simulink model "gm_interlock_deadtime"  (R2020b)
settings: Solver=FixedStepDiscrete  StartTime=0.0  StopTime=0.01  RelTol=1e-3
libraries: hdlmdlgenlib x12, simulink x6, hdlsllib x6, eePwmGeneratorTwoLevel x1, powerlib_meascontrol x1
settings Model: Creator=ts  LastModifiedBy=ts
settings DataIOCC: LimitDataPoints=on  SaveOutput=off  SaveTime=off
settings OptimizationCC: BlockReduction=off  ConditionallyExecuteInputs=off  DefaultParameterBehavior=Inlined  LifeSpan=inf
settings DebuggingCC: AlgebraicLoopMsg=error  InheritedTsInSrcMsg=none  SingleTaskRateTransMsg=error  AllowSymbolicDim=off  StrictBusMsg=ErrorOnBusTreatedAsVector  SFUnexpectedBacktrackingDiag=warning  SFNoUnconditionalDefaultTransitionDiag=warning  SFExecutionAtInitializationDiag=none  ArithmeticOperatorsInVariantConditions=warning
settings HardwareCC: ProdBitPerPointer=32  ProdBitPerSizeT=32  ProdBitPerPtrDiffT=32  ProdLargestAtomicFloat=None  ProdIntDivRoundTo=Undefined  ProdEndianess=Unspecified  ProdWordSize=32  ProdHWDeviceType=ASIC/FPGA->ASIC/FPGA  ProdEqTarget=off
settings SFSimCC: SimUseLocalCustomCode=off  CustomCodeUndefinedFunction=UseInterfaceOnly
settings RTWCC: RTWUseLocalCustomCode=off
settings CodeAppCC: StateflowObjectComments=on
settings GRTTargetCC: TargetLangStandard=C89/C90 (ANSI)
settings ConfigComp: CovScope=ReferencedModels  CovMetricSettings=dw  CovSaveCumulativeToWorkspaceVar=on  CovSaveSingleToWorkspaceVar=on  CovExternalEMLEnable=off  CovSFcnEnable=off

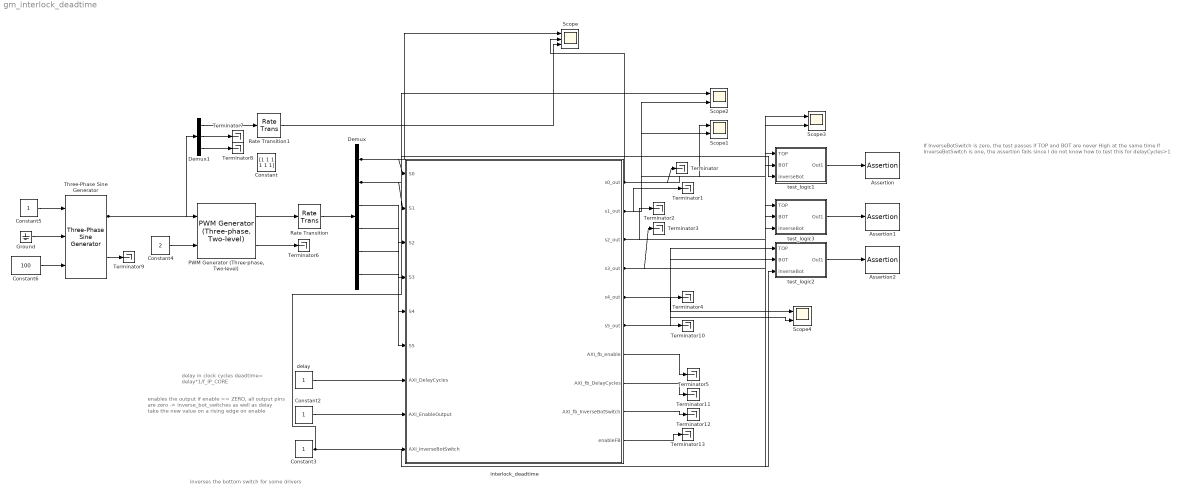
== system gm_interlock_deadtime ==
  note: delay in clock cycles
      | deadtime= delay*1/f_IP_CORE
  note: inverses the bottom switch for some drivers
  note: enables the output
      | if enable == ZERO, all output pins are zero
      |
      | -> inverse_bot_switches as well as delay take the
      | new value on a rising edge on enable
  note: If InverseBotSwitch is zero, the test passes if TOP and BOT are never High at the same time
      | If InverseBotSwitch is one, the assertion fails since I do not know how to test this for delayCycles>1
  Assertion : Assertion
  Assertion1 : Assertion
  Assertion2 : Assertion
  Constant : Constant  Value=[1 1 1 1 1 1]  OutDataTypeStr=boolean
  Constant2 : Constant  OutDataTypeStr=boolean  SampleTime=1/100e6
  Constant3 : Constant  OutDataTypeStr=boolean  SampleTime=1/100e6
  Constant4 : Constant  Value=2  SampleTime=-1
  Constant5 : Constant  SampleTime=-1
  Constant6 : Constant  Value=100  SampleTime=-1
  Demux : Demux  Outputs=6
  Demux1 : Demux  Outputs=3
  Ground : Ground
  "PWM Generator (Three-phase, Two-level)" : eePwmGeneratorTwoLevel/PWM Generator (Three-phase, Two-level)  PWMMode=Continuous PWM (CPWM)  CPWMMode=SPWM: sinusoidal PWM  DPWMMode=60 DPWM: 60 degree discontinuous PWM  fsw=10e3  Ts=1/(100*100e3)
      settings: SourceProductBaseCode=PS
  Rate Transition : RateTransition  OutPortSampleTime=1/100e6
  Rate Transition1 : RateTransition  OutPortSampleTime=1/100e6
  Scope : Scope  NumInputPorts=3
  Scope{1..4} (4 alike) : Scope  NumInputPorts=2
  Terminator{,1..13} (14 alike) : Terminator
  Three-Phase Sine Generator : powerlib_meascontrol/Pulse & Signal Generators/Three-Phase Sine Generator  Ts=1/100e3
      settings: SourceProductBaseCode=PS
  delay : Constant  OutDataTypeStr=fixdt(0,10,0)  SampleTime=1/100e6
  interlock_deadtime : Subsystem  TreatAsAtomicUnit=on
  test_logic1 : Subsystem
  test_logic2 : Subsystem
  test_logic3 : Subsystem
  wires:
  delay/1 -> interlock_deadtime/7(AXI_DelayCycles)
  "PWM Generator (Three-phase, Two-level)"/1 -> Rate Transition/1
  Rate Transition/1 -> Demux/1
  test_logic1/1(Out1) -> Assertion/1
  test_logic2/1(Out1) -> Assertion2/1
  test_logic3/1(Out1) -> Assertion1/1
  interlock_deadtime/10(enableFB) -> Terminator13/1
  interlock_deadtime/9(AXI_fb_InverseBotSwitch) -> Terminator12/1
  interlock_deadtime/8(AXI_fb_DelayCycles) -> Terminator11/1
  interlock_deadtime/7(AXI_fb_enable) -> Terminator5/1
  interlock_deadtime/6(s5_out) -> Terminator10/1, test_logic2/2(BOT), Scope4/2
  Ground/1 -> Three-Phase Sine Generator/2
  Three-Phase Sine Generator/2 -> Terminator9/1
  Demux1/3 -> Terminator8/1
  Demux1/2 -> Terminator7/1
  "PWM Generator (Three-phase, Two-level)"/2 -> Terminator6/1
  Constant3/1 -> test_logic1/3(inverseBot), test_logic3/3(inverseBot), test_logic2/3(inverseBot), interlock_deadtime/9(AXI_InverseBotSwitch)
  Rate Transition1/1 -> Scope/3
  Demux1/1 -> Rate Transition1/1
  Demux/6 -> interlock_deadtime/6(S5)
  Demux/5 -> interlock_deadtime/5(S4)
  Demux/4 -> interlock_deadtime/4(S3)
  Demux/3 -> interlock_deadtime/3(S2)
  Demux/2 -> interlock_deadtime/2(S1), Scope2/1
  Demux/1 -> interlock_deadtime/1(S0), Scope/1
  Constant6/1 -> Three-Phase Sine Generator/3
  Constant5/1 -> Three-Phase Sine Generator/1
  Three-Phase Sine Generator/1 -> "PWM Generator (Three-phase, Two-level)"/1, Demux1/1
  Constant4/1 -> "PWM Generator (Three-phase, Two-level)"/2
  interlock_deadtime/5(s4_out) -> Terminator4/1, test_logic2/1(TOP), Scope4/1
  interlock_deadtime/4(s3_out) -> Terminator3/1, test_logic3/2(BOT), Scope3/2
  interlock_deadtime/3(s2_out) -> Terminator2/1, test_logic3/1(TOP), Scope3/1
  interlock_deadtime/2(s1_out) -> Terminator1/1, test_logic1/2(BOT), Scope2/2, Scope1/2
  interlock_deadtime/1(s0_out) -> Scope1/1, Terminator/1, test_logic1/1(TOP), Scope/2
  Constant2/1 -> interlock_deadtime/8(AXI_EnableOutput)

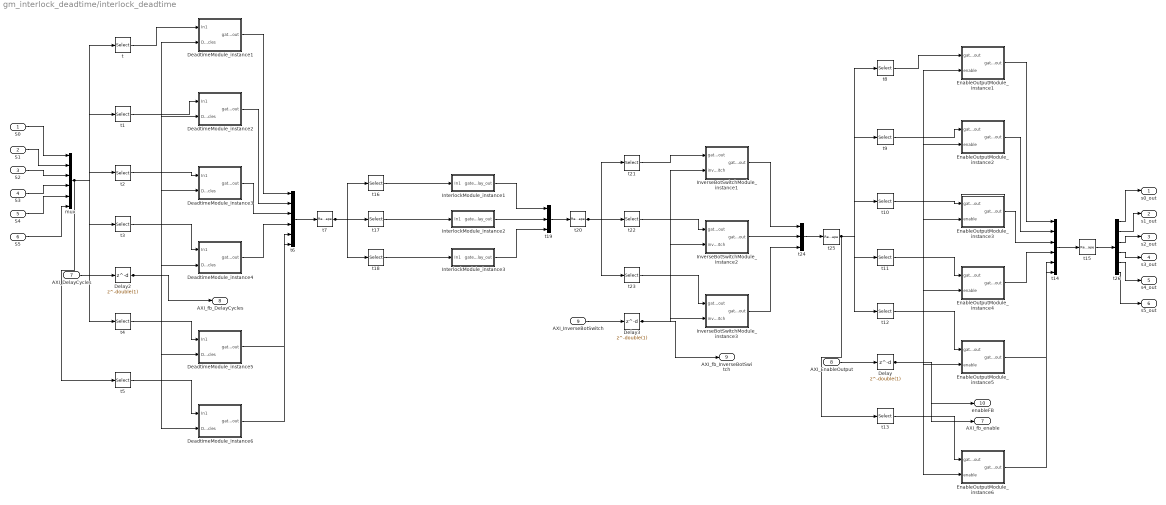
== system gm_interlock_deadtime/interlock_deadtime ==
  S0 : Inport  OutDataTypeStr=boolean  PortDimensions=1  SampleTime=1e-08
  S1 : Inport  Port=2  OutDataTypeStr=boolean  PortDimensions=1  SampleTime=1e-08
  S2 : Inport  Port=3  OutDataTypeStr=boolean  PortDimensions=1  SampleTime=1e-08
  S3 : Inport  Port=4  OutDataTypeStr=boolean  PortDimensions=1  SampleTime=1e-08
  S4 : Inport  Port=5  OutDataTypeStr=boolean  PortDimensions=1  SampleTime=1e-08
  S5 : Inport  Port=6  OutDataTypeStr=boolean  PortDimensions=1  SampleTime=1e-08
  AXI_DelayCycles : Inport  Port=7  OutDataTypeStr=fixdt(0, 10, 0)  PortDimensions=1  SampleTime=1e-08
  AXI_EnableOutput : Inport  Port=8  OutDataTypeStr=boolean  PortDimensions=1  SampleTime=1e-08
  AXI_InverseBotSwitch : Inport  Port=9  OutDataTypeStr=boolean  PortDimensions=1  SampleTime=1e-08
  DeadtimeModule_instance1 : Subsystem
  DeadtimeModule_instance2 : Subsystem
  DeadtimeModule_instance3 : Subsystem
  DeadtimeModule_instance4 : Subsystem
  DeadtimeModule_instance5 : Subsystem
  DeadtimeModule_instance6 : Subsystem
  Delay : Delay  DelayLength=double(1)  InitialCondition=0  SampleTime=1e-08
  Delay2 : Delay  DelayLength=double(1)  InitialCondition=0  SampleTime=1e-08
  Delay3 : Delay  DelayLength=double(1)  InitialCondition=0  SampleTime=1e-08
  EnableOutputModule_instance1 : Subsystem
  EnableOutputModule_instance2 : Subsystem
  EnableOutputModule_instance3 : Subsystem
  EnableOutputModule_instance4 : Subsystem
  EnableOutputModule_instance5 : Subsystem
  EnableOutputModule_instance6 : Subsystem
  InterlockModule_instance1 : Subsystem
  InterlockModule_instance2 : Subsystem
  InterlockModule_instance3 : Subsystem
  InverseBotSwitchModule_instance1 : Subsystem
  InverseBotSwitchModule_instance2 : Subsystem
  InverseBotSwitchModule_instance3 : Subsystem
  mux : Mux  Inputs=6
  t : Selector  SampleTime=1e-08  IndexOptions=Index vector (dialog)  Indices=double(1)  OutputSizes=1
  t1 : Selector  SampleTime=1e-08  IndexOptions=Index vector (dialog)  Indices=double(2)  OutputSizes=1
  t10 : Selector  SampleTime=1e-08  IndexOptions=Index vector (dialog)  Indices=double(3)  OutputSizes=1
  t11 : Selector  SampleTime=1e-08  IndexOptions=Index vector (dialog)  Indices=double(4)  OutputSizes=1
  t12 : Selector  SampleTime=1e-08  IndexOptions=Index vector (dialog)  Indices=double(5)  OutputSizes=1
  t13 : Selector  SampleTime=1e-08  IndexOptions=Index vector (dialog)  Indices=double(6)  OutputSizes=1
  t14 : Concatenate  NumInputs=6
  t{7,15,20,25} (4 alike) : Reshape
  t16 : Selector  SampleTime=1e-08  IndexOptions=Index vector (dialog)  Indices=double([1 2])  OutputSizes=1
  t17 : Selector  SampleTime=1e-08  IndexOptions=Index vector (dialog)  Indices=double([3 4])  OutputSizes=1
  t18 : Selector  SampleTime=1e-08  IndexOptions=Index vector (dialog)  Indices=double([5 6])  OutputSizes=1
  t19 : Concatenate  NumInputs=3
  t2 : Selector  SampleTime=1e-08  IndexOptions=Index vector (dialog)  Indices=double(3)  OutputSizes=1
  t21 : Selector  SampleTime=1e-08  IndexOptions=Index vector (dialog)  Indices=double([1 2])  OutputSizes=1
  t22 : Selector  SampleTime=1e-08  IndexOptions=Index vector (dialog)  Indices=double([3 4])  OutputSizes=1
  t23 : Selector  SampleTime=1e-08  IndexOptions=Index vector (dialog)  Indices=double([5 6])  OutputSizes=1
  t24 : Concatenate  NumInputs=3
  t26 : Demux  Outputs=6
  t3 : Selector  SampleTime=1e-08  IndexOptions=Index vector (dialog)  Indices=double(4)  OutputSizes=1
  t4 : Selector  SampleTime=1e-08  IndexOptions=Index vector (dialog)  Indices=double(5)  OutputSizes=1
  t5 : Selector  SampleTime=1e-08  IndexOptions=Index vector (dialog)  Indices=double(6)  OutputSizes=1
  t6 : Concatenate  NumInputs=6
  t8 : Selector  SampleTime=1e-08  IndexOptions=Index vector (dialog)  Indices=double(1)  OutputSizes=1
  t9 : Selector  SampleTime=1e-08  IndexOptions=Index vector (dialog)  Indices=double(2)  OutputSizes=1
  s0_out : Outport  VectorParamsAs1DForOutWhenUnconnected=off
  s1_out : Outport  Port=2  VectorParamsAs1DForOutWhenUnconnected=off
  s2_out : Outport  Port=3  VectorParamsAs1DForOutWhenUnconnected=off
  s3_out : Outport  Port=4  VectorParamsAs1DForOutWhenUnconnected=off
  s4_out : Outport  Port=5  VectorParamsAs1DForOutWhenUnconnected=off
  s5_out : Outport  Port=6  VectorParamsAs1DForOutWhenUnconnected=off
  AXI_fb_enable : Outport  Port=7  VectorParamsAs1DForOutWhenUnconnected=off
  AXI_fb_DelayCycles : Outport  Port=8  VectorParamsAs1DForOutWhenUnconnected=off
  AXI_fb_InverseBotSwitch : Outport  Port=9  VectorParamsAs1DForOutWhenUnconnected=off
  enableFB : Outport  Port=10  VectorParamsAs1DForOutWhenUnconnected=off
  wires:
  S0/1 -> mux/1
  S1/1 -> mux/2
  S2/1 -> mux/3
  S3/1 -> mux/4
  S4/1 -> mux/5
  S5/1 -> mux/6
  AXI_DelayCycles/1 -> Delay2/1
  AXI_EnableOutput/1 -> Delay/1
  AXI_InverseBotSwitch/1 -> Delay3/1
  t7/1 -> t18/1, t17/1, t16/1
  Delay/1 -> EnableOutputModule_instance6/2(enable), EnableOutputModule_instance5/2(enable), EnableOutputModule_instance4/2(enable), EnableOutputModule_instance3/2(enable), EnableOutputModule_instance2/2(enable), EnableOutputModule_instance1/2(enable), AXI_fb_enable/1, enableFB/1
  Delay2/1 -> DeadtimeModule_instance6/2(DelayCycles), DeadtimeModule_instance5/2(DelayCycles), DeadtimeModule_instance4/2(DelayCycles), DeadtimeModule_instance3/2(DelayCycles), DeadtimeModule_instance2/2(DelayCycles), DeadtimeModule_instance1/2(DelayCycles), AXI_fb_DelayCycles/1
  Delay3/1 -> InverseBotSwitchModule_instance3/2(inverse_bottom_switch), InverseBotSwitchModule_instance2/2(inverse_bottom_switch), InverseBotSwitchModule_instance1/2(inverse_bottom_switch), AXI_fb_InverseBotSwitch/1
  t15/1 -> t26/1
  t20/1 -> t23/1, t22/1, t21/1
  t25/1 -> t13/1, t12/1, t11/1, t10/1, t9/1, t8/1
  mux/1 -> t5/1, t4/1, t3/1, t2/1, t1/1, t/1
  t/1 -> DeadtimeModule_instance1/1(In1)
  t1/1 -> DeadtimeModule_instance2/1(In1)
  t2/1 -> DeadtimeModule_instance3/1(In1)
  t3/1 -> DeadtimeModule_instance4/1(In1)
  t4/1 -> DeadtimeModule_instance5/1(In1)
  t5/1 -> DeadtimeModule_instance6/1(In1)
  t6/1 -> t7/1
  DeadtimeModule_instance1/1(gate_delay_out) -> t6/1
  DeadtimeModule_instance2/1(gate_delay_out) -> t6/2
  DeadtimeModule_instance3/1(gate_delay_out) -> t6/3
  DeadtimeModule_instance4/1(gate_delay_out) -> t6/4
  DeadtimeModule_instance5/1(gate_delay_out) -> t6/5
  DeadtimeModule_instance6/1(gate_delay_out) -> t6/6
  t8/1 -> EnableOutputModule_instance1/1(gate_delay_out)
  t9/1 -> EnableOutputModule_instance2/1(gate_delay_out)
  t10/1 -> EnableOutputModule_instance3/1(gate_delay_out)
  t11/1 -> EnableOutputModule_instance4/1(gate_delay_out)
  t12/1 -> EnableOutputModule_instance5/1(gate_delay_out)
  t13/1 -> EnableOutputModule_instance6/1(gate_delay_out)
  t14/1 -> t15/1
  EnableOutputModule_instance1/1(gate_enable_out) -> t14/1
  EnableOutputModule_instance2/1(gate_enable_out) -> t14/2
  EnableOutputModule_instance3/1(gate_enable_out) -> t14/3
  EnableOutputModule_instance4/1(gate_enable_out) -> t14/4
  EnableOutputModule_instance5/1(gate_enable_out) -> t14/5
  EnableOutputModule_instance6/1(gate_enable_out) -> t14/6
  t16/1 -> InterlockModule_instance1/1(In1)
  t17/1 -> InterlockModule_instance2/1(In1)
  t18/1 -> InterlockModule_instance3/1(In1)
  t19/1 -> t20/1
  InterlockModule_instance1/1(gate_delay_out) -> t19/1
  InterlockModule_instance2/1(gate_delay_out) -> t19/2
  InterlockModule_instance3/1(gate_delay_out) -> t19/3
  t21/1 -> InverseBotSwitchModule_instance1/1(gate_delay_out)
  t22/1 -> InverseBotSwitchModule_instance2/1(gate_delay_out)
  t23/1 -> InverseBotSwitchModule_instance3/1(gate_delay_out)
  t24/1 -> t25/1
  InverseBotSwitchModule_instance1/1(gate_enable_out) -> t24/1
  InverseBotSwitchModule_instance2/1(gate_enable_out) -> t24/2
  InverseBotSwitchModule_instance3/1(gate_enable_out) -> t24/3
  t26/1 -> s0_out/1
  t26/2 -> s1_out/1
  t26/3 -> s2_out/1
  t26/4 -> s3_out/1
  t26/5 -> s4_out/1
  t26/6 -> s5_out/1

== system gm_interlock_deadtime/test_logic1 ==
  TOP : Inport
  BOT : Inport  Port=2
  inverseBot : Inport  Port=3
  AND : Logic  IconShape=distinctive  AllPortsSameDT=off  OutDataTypeStr=boolean
  Constant : Constant
  NOT : Logic  Operator=NOT  IconShape=distinctive  AllPortsSameDT=off  OutDataTypeStr=boolean
  Switch : Switch  Criteria=u2 ~= 0
  Out1 : Outport
  wires:
  BOT/1 -> AND/2
  TOP/1 -> AND/1
  NOT/1 -> Switch/3
  inverseBot/1 -> Switch/2
  AND/1 -> NOT/1
  Switch/1 -> Out1/1
  Constant/1 -> Switch/1

== system gm_interlock_deadtime/test_logic2 ==
  TOP : Inport
  BOT : Inport  Port=2
  inverseBot : Inport  Port=3
  AND : Logic  IconShape=distinctive  AllPortsSameDT=off  OutDataTypeStr=boolean
  Constant : Constant
  NOT : Logic  Operator=NOT  IconShape=distinctive  AllPortsSameDT=off  OutDataTypeStr=boolean
  Switch : Switch  Criteria=u2 ~= 0
  Out1 : Outport
  wires:
  Constant/1 -> Switch/1
  Switch/1 -> Out1/1
  AND/1 -> NOT/1
  inverseBot/1 -> Switch/2
  NOT/1 -> Switch/3
  TOP/1 -> AND/1
  BOT/1 -> AND/2

== system gm_interlock_deadtime/test_logic3 ==
  TOP : Inport
  BOT : Inport  Port=2
  inverseBot : Inport  Port=3
  AND : Logic  IconShape=distinctive  AllPortsSameDT=off  OutDataTypeStr=boolean
  Constant : Constant
  NOT : Logic  Operator=NOT  IconShape=distinctive  AllPortsSameDT=off  OutDataTypeStr=boolean
  Switch : Switch  Criteria=u2 ~= 0
  Out1 : Outport
  wires:
  BOT/1 -> AND/2
  TOP/1 -> AND/1
  NOT/1 -> Switch/3
  inverseBot/1 -> Switch/2
  AND/1 -> NOT/1
  Switch/1 -> Out1/1
  Constant/1 -> Switch/1

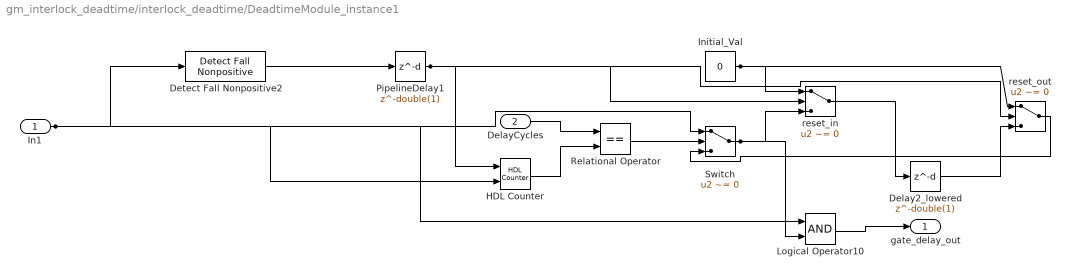
== system gm_interlock_deadtime/interlock_deadtime/DeadtimeModule_instance1 ==
  In1 : Inport  OutDataTypeStr=boolean  PortDimensions=1  SampleTime=1e-08
  DelayCycles : Inport  Port=2  OutDataTypeStr=fixdt(0, 10, 0)  PortDimensions=1  SampleTime=1e-08
  Delay2_lowered : Delay  DelayLength=double(1)  InitialCondition=0  SampleTime=1e-08
  Detect Fall Nonpositive2 : simulink/Logic and Bit Operations/Detect Fall Nonpositive  vinit=0  OutDataTypeStr=boolean
      settings: SourceProductBaseCode=SL
  HDL Counter : hdlsllib/Sources/HDL Counter  CountType=Free running  CountInit=double(0)  CountStep=double(1)  CountMax=25  CountFromType=Initial value  CountFrom=double(0)  CountResetPort=on  CountLoadPort=off  CountEnbPort=on  CountDirPort=off  CountDataType=Unsigned  CountWordLen=10  CountFracLen=0  CountSampTime=1e-08
  Initial_Val : Constant  Value=0  OutDataTypeStr=boolean  SampleTime=1e-08
  Logical Operator10 : Logic  AllPortsSameDT=off  OutDataTypeStr=boolean  SampleTime=1e-08
  PipelineDelay1 : Delay  DelayLength=double(1)  InitialCondition=0  SampleTime=1e-08
  Relational Operator : RelationalOperator  Operator===  OutDataTypeStr=boolean  SampleTime=1e-08  RndMeth=Nearest
  Switch : Switch  Criteria=u2 ~= 0  Threshold=double(0)  OutDataTypeStr=boolean  SampleTime=1e-08
  reset_in : Switch  Criteria=u2 ~= 0  Threshold=double(0)  OutDataTypeStr=boolean  SampleTime=1e-08
  reset_out : Switch  Criteria=u2 ~= 0  Threshold=double(0)  OutDataTypeStr=boolean  SampleTime=1e-08
  gate_delay_out : Outport
  wires:
  In1/1 -> Logical Operator10/1, Switch/1, HDL Counter/2, Detect Fall Nonpositive2/1
  DelayCycles/1 -> Relational Operator/1
  Switch/1 -> Logical Operator10/2, reset_in/3
  Relational Operator/1 -> Switch/2
  PipelineDelay1/1 -> reset_out/2, reset_in/2, HDL Counter/1
  Logical Operator10/1 -> gate_delay_out/1
  HDL Counter/1 -> Relational Operator/2
  Detect Fall Nonpositive2/1 -> PipelineDelay1/1
  reset_out/1 -> Switch/3
  Initial_Val/1 -> reset_out/1, reset_in/1
  Delay2_lowered/1 -> reset_out/3
  reset_in/1 -> Delay2_lowered/1

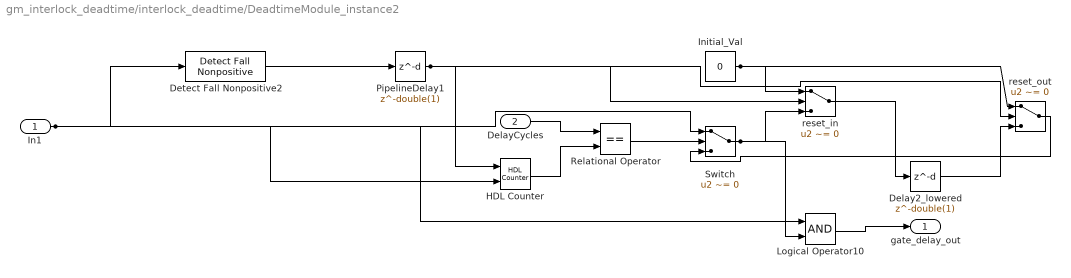
== system gm_interlock_deadtime/interlock_deadtime/DeadtimeModule_instance2 ==
  In1 : Inport  OutDataTypeStr=boolean  PortDimensions=1  SampleTime=1e-08
  DelayCycles : Inport  Port=2  OutDataTypeStr=fixdt(0, 10, 0)  PortDimensions=1  SampleTime=1e-08
  Delay2_lowered : Delay  DelayLength=double(1)  InitialCondition=0  SampleTime=1e-08
  Detect Fall Nonpositive2 : simulink/Logic and Bit Operations/Detect Fall Nonpositive  vinit=0  OutDataTypeStr=boolean
      settings: SourceProductBaseCode=SL
  HDL Counter : hdlsllib/Sources/HDL Counter  CountType=Free running  CountInit=double(0)  CountStep=double(1)  CountMax=25  CountFromType=Initial value  CountFrom=double(0)  CountResetPort=on  CountLoadPort=off  CountEnbPort=on  CountDirPort=off  CountDataType=Unsigned  CountWordLen=10  CountFracLen=0  CountSampTime=1e-08
  Initial_Val : Constant  Value=0  OutDataTypeStr=boolean  SampleTime=1e-08
  Logical Operator10 : Logic  AllPortsSameDT=off  OutDataTypeStr=boolean  SampleTime=1e-08
  PipelineDelay1 : Delay  DelayLength=double(1)  InitialCondition=0  SampleTime=1e-08
  Relational Operator : RelationalOperator  Operator===  OutDataTypeStr=boolean  SampleTime=1e-08  RndMeth=Nearest
  Switch : Switch  Criteria=u2 ~= 0  Threshold=double(0)  OutDataTypeStr=boolean  SampleTime=1e-08
  reset_in : Switch  Criteria=u2 ~= 0  Threshold=double(0)  OutDataTypeStr=boolean  SampleTime=1e-08
  reset_out : Switch  Criteria=u2 ~= 0  Threshold=double(0)  OutDataTypeStr=boolean  SampleTime=1e-08
  gate_delay_out : Outport
  wires:
  reset_in/1 -> Delay2_lowered/1
  Delay2_lowered/1 -> reset_out/3
  Initial_Val/1 -> reset_in/1, reset_out/1
  reset_out/1 -> Switch/3
  Detect Fall Nonpositive2/1 -> PipelineDelay1/1
  HDL Counter/1 -> Relational Operator/2
  Logical Operator10/1 -> gate_delay_out/1
  PipelineDelay1/1 -> HDL Counter/1, reset_in/2, reset_out/2
  Relational Operator/1 -> Switch/2
  Switch/1 -> reset_in/3, Logical Operator10/2
  DelayCycles/1 -> Relational Operator/1
  In1/1 -> Detect Fall Nonpositive2/1, HDL Counter/2, Switch/1, Logical Operator10/1

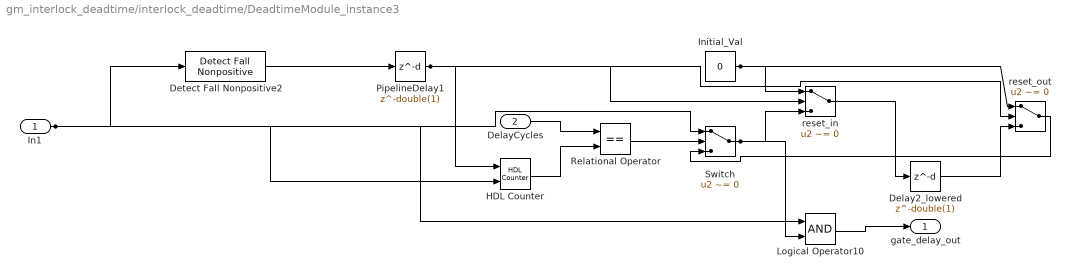
== system gm_interlock_deadtime/interlock_deadtime/DeadtimeModule_instance3 ==
  In1 : Inport  OutDataTypeStr=boolean  PortDimensions=1  SampleTime=1e-08
  DelayCycles : Inport  Port=2  OutDataTypeStr=fixdt(0, 10, 0)  PortDimensions=1  SampleTime=1e-08
  Delay2_lowered : Delay  DelayLength=double(1)  InitialCondition=0  SampleTime=1e-08
  Detect Fall Nonpositive2 : simulink/Logic and Bit Operations/Detect Fall Nonpositive  vinit=0  OutDataTypeStr=boolean
      settings: SourceProductBaseCode=SL
  HDL Counter : hdlsllib/Sources/HDL Counter  CountType=Free running  CountInit=double(0)  CountStep=double(1)  CountMax=25  CountFromType=Initial value  CountFrom=double(0)  CountResetPort=on  CountLoadPort=off  CountEnbPort=on  CountDirPort=off  CountDataType=Unsigned  CountWordLen=10  CountFracLen=0  CountSampTime=1e-08
  Initial_Val : Constant  Value=0  OutDataTypeStr=boolean  SampleTime=1e-08
  Logical Operator10 : Logic  AllPortsSameDT=off  OutDataTypeStr=boolean  SampleTime=1e-08
  PipelineDelay1 : Delay  DelayLength=double(1)  InitialCondition=0  SampleTime=1e-08
  Relational Operator : RelationalOperator  Operator===  OutDataTypeStr=boolean  SampleTime=1e-08  RndMeth=Nearest
  Switch : Switch  Criteria=u2 ~= 0  Threshold=double(0)  OutDataTypeStr=boolean  SampleTime=1e-08
  reset_in : Switch  Criteria=u2 ~= 0  Threshold=double(0)  OutDataTypeStr=boolean  SampleTime=1e-08
  reset_out : Switch  Criteria=u2 ~= 0  Threshold=double(0)  OutDataTypeStr=boolean  SampleTime=1e-08
  gate_delay_out : Outport
  wires:
  reset_in/1 -> Delay2_lowered/1
  Delay2_lowered/1 -> reset_out/3
  Initial_Val/1 -> reset_in/1, reset_out/1
  reset_out/1 -> Switch/3
  Detect Fall Nonpositive2/1 -> PipelineDelay1/1
  HDL Counter/1 -> Relational Operator/2
  Logical Operator10/1 -> gate_delay_out/1
  PipelineDelay1/1 -> HDL Counter/1, reset_in/2, reset_out/2
  Relational Operator/1 -> Switch/2
  Switch/1 -> reset_in/3, Logical Operator10/2
  DelayCycles/1 -> Relational Operator/1
  In1/1 -> Detect Fall Nonpositive2/1, HDL Counter/2, Switch/1, Logical Operator10/1

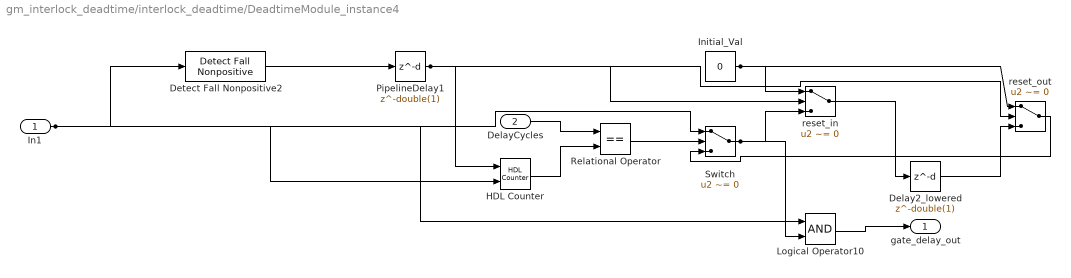
== system gm_interlock_deadtime/interlock_deadtime/DeadtimeModule_instance4 ==
  In1 : Inport  OutDataTypeStr=boolean  PortDimensions=1  SampleTime=1e-08
  DelayCycles : Inport  Port=2  OutDataTypeStr=fixdt(0, 10, 0)  PortDimensions=1  SampleTime=1e-08
  Delay2_lowered : Delay  DelayLength=double(1)  InitialCondition=0  SampleTime=1e-08
  Detect Fall Nonpositive2 : simulink/Logic and Bit Operations/Detect Fall Nonpositive  vinit=0  OutDataTypeStr=boolean
      settings: SourceProductBaseCode=SL
  HDL Counter : hdlsllib/Sources/HDL Counter  CountType=Free running  CountInit=double(0)  CountStep=double(1)  CountMax=25  CountFromType=Initial value  CountFrom=double(0)  CountResetPort=on  CountLoadPort=off  CountEnbPort=on  CountDirPort=off  CountDataType=Unsigned  CountWordLen=10  CountFracLen=0  CountSampTime=1e-08
  Initial_Val : Constant  Value=0  OutDataTypeStr=boolean  SampleTime=1e-08
  Logical Operator10 : Logic  AllPortsSameDT=off  OutDataTypeStr=boolean  SampleTime=1e-08
  PipelineDelay1 : Delay  DelayLength=double(1)  InitialCondition=0  SampleTime=1e-08
  Relational Operator : RelationalOperator  Operator===  OutDataTypeStr=boolean  SampleTime=1e-08  RndMeth=Nearest
  Switch : Switch  Criteria=u2 ~= 0  Threshold=double(0)  OutDataTypeStr=boolean  SampleTime=1e-08
  reset_in : Switch  Criteria=u2 ~= 0  Threshold=double(0)  OutDataTypeStr=boolean  SampleTime=1e-08
  reset_out : Switch  Criteria=u2 ~= 0  Threshold=double(0)  OutDataTypeStr=boolean  SampleTime=1e-08
  gate_delay_out : Outport
  wires:
  reset_in/1 -> Delay2_lowered/1
  Delay2_lowered/1 -> reset_out/3
  Initial_Val/1 -> reset_in/1, reset_out/1
  reset_out/1 -> Switch/3
  Detect Fall Nonpositive2/1 -> PipelineDelay1/1
  HDL Counter/1 -> Relational Operator/2
  Logical Operator10/1 -> gate_delay_out/1
  PipelineDelay1/1 -> HDL Counter/1, reset_in/2, reset_out/2
  Relational Operator/1 -> Switch/2
  Switch/1 -> reset_in/3, Logical Operator10/2
  DelayCycles/1 -> Relational Operator/1
  In1/1 -> Detect Fall Nonpositive2/1, HDL Counter/2, Switch/1, Logical Operator10/1

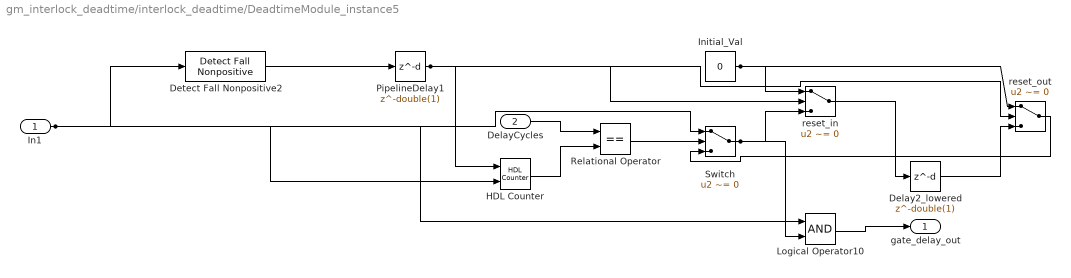
== system gm_interlock_deadtime/interlock_deadtime/DeadtimeModule_instance5 ==
  In1 : Inport  OutDataTypeStr=boolean  PortDimensions=1  SampleTime=1e-08
  DelayCycles : Inport  Port=2  OutDataTypeStr=fixdt(0, 10, 0)  PortDimensions=1  SampleTime=1e-08
  Delay2_lowered : Delay  DelayLength=double(1)  InitialCondition=0  SampleTime=1e-08
  Detect Fall Nonpositive2 : simulink/Logic and Bit Operations/Detect Fall Nonpositive  vinit=0  OutDataTypeStr=boolean
      settings: SourceProductBaseCode=SL
  HDL Counter : hdlsllib/Sources/HDL Counter  CountType=Free running  CountInit=double(0)  CountStep=double(1)  CountMax=25  CountFromType=Initial value  CountFrom=double(0)  CountResetPort=on  CountLoadPort=off  CountEnbPort=on  CountDirPort=off  CountDataType=Unsigned  CountWordLen=10  CountFracLen=0  CountSampTime=1e-08
  Initial_Val : Constant  Value=0  OutDataTypeStr=boolean  SampleTime=1e-08
  Logical Operator10 : Logic  AllPortsSameDT=off  OutDataTypeStr=boolean  SampleTime=1e-08
  PipelineDelay1 : Delay  DelayLength=double(1)  InitialCondition=0  SampleTime=1e-08
  Relational Operator : RelationalOperator  Operator===  OutDataTypeStr=boolean  SampleTime=1e-08  RndMeth=Nearest
  Switch : Switch  Criteria=u2 ~= 0  Threshold=double(0)  OutDataTypeStr=boolean  SampleTime=1e-08
  reset_in : Switch  Criteria=u2 ~= 0  Threshold=double(0)  OutDataTypeStr=boolean  SampleTime=1e-08
  reset_out : Switch  Criteria=u2 ~= 0  Threshold=double(0)  OutDataTypeStr=boolean  SampleTime=1e-08
  gate_delay_out : Outport
  wires:
  reset_in/1 -> Delay2_lowered/1
  Delay2_lowered/1 -> reset_out/3
  Initial_Val/1 -> reset_in/1, reset_out/1
  reset_out/1 -> Switch/3
  Detect Fall Nonpositive2/1 -> PipelineDelay1/1
  HDL Counter/1 -> Relational Operator/2
  Logical Operator10/1 -> gate_delay_out/1
  PipelineDelay1/1 -> HDL Counter/1, reset_in/2, reset_out/2
  Relational Operator/1 -> Switch/2
  Switch/1 -> reset_in/3, Logical Operator10/2
  DelayCycles/1 -> Relational Operator/1
  In1/1 -> Detect Fall Nonpositive2/1, HDL Counter/2, Switch/1, Logical Operator10/1

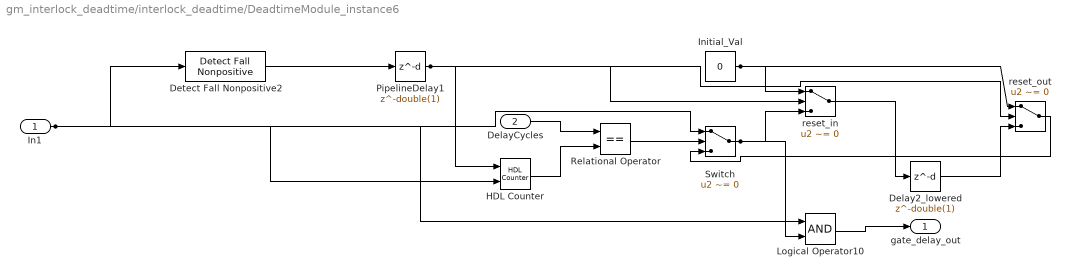
== system gm_interlock_deadtime/interlock_deadtime/DeadtimeModule_instance6 ==
  In1 : Inport  OutDataTypeStr=boolean  PortDimensions=1  SampleTime=1e-08
  DelayCycles : Inport  Port=2  OutDataTypeStr=fixdt(0, 10, 0)  PortDimensions=1  SampleTime=1e-08
  Delay2_lowered : Delay  DelayLength=double(1)  InitialCondition=0  SampleTime=1e-08
  Detect Fall Nonpositive2 : simulink/Logic and Bit Operations/Detect Fall Nonpositive  vinit=0  OutDataTypeStr=boolean
      settings: SourceProductBaseCode=SL
  HDL Counter : hdlsllib/Sources/HDL Counter  CountType=Free running  CountInit=double(0)  CountStep=double(1)  CountMax=25  CountFromType=Initial value  CountFrom=double(0)  CountResetPort=on  CountLoadPort=off  CountEnbPort=on  CountDirPort=off  CountDataType=Unsigned  CountWordLen=10  CountFracLen=0  CountSampTime=1e-08
  Initial_Val : Constant  Value=0  OutDataTypeStr=boolean  SampleTime=1e-08
  Logical Operator10 : Logic  AllPortsSameDT=off  OutDataTypeStr=boolean  SampleTime=1e-08
  PipelineDelay1 : Delay  DelayLength=double(1)  InitialCondition=0  SampleTime=1e-08
  Relational Operator : RelationalOperator  Operator===  OutDataTypeStr=boolean  SampleTime=1e-08  RndMeth=Nearest
  Switch : Switch  Criteria=u2 ~= 0  Threshold=double(0)  OutDataTypeStr=boolean  SampleTime=1e-08
  reset_in : Switch  Criteria=u2 ~= 0  Threshold=double(0)  OutDataTypeStr=boolean  SampleTime=1e-08
  reset_out : Switch  Criteria=u2 ~= 0  Threshold=double(0)  OutDataTypeStr=boolean  SampleTime=1e-08
  gate_delay_out : Outport
  wires:
  reset_in/1 -> Delay2_lowered/1
  Delay2_lowered/1 -> reset_out/3
  Initial_Val/1 -> reset_in/1, reset_out/1
  reset_out/1 -> Switch/3
  Detect Fall Nonpositive2/1 -> PipelineDelay1/1
  HDL Counter/1 -> Relational Operator/2
  Logical Operator10/1 -> gate_delay_out/1
  PipelineDelay1/1 -> HDL Counter/1, reset_in/2, reset_out/2
  Relational Operator/1 -> Switch/2
  Switch/1 -> reset_in/3, Logical Operator10/2
  DelayCycles/1 -> Relational Operator/1
  In1/1 -> Detect Fall Nonpositive2/1, HDL Counter/2, Switch/1, Logical Operator10/1

== system gm_interlock_deadtime/interlock_deadtime/EnableOutputModule_instance1 ==
  gate_delay_out : Inport  OutDataTypeStr=boolean  PortDimensions=1  SampleTime=1e-08
  enable : Inport  Port=2  OutDataTypeStr=boolean  PortDimensions=1  SampleTime=1e-08
  AND : Logic  AllPortsSameDT=off  OutDataTypeStr=boolean  SampleTime=1e-08
  gate_enable_out : Outport
  wires:
  gate_delay_out/1 -> AND/1
  enable/1 -> AND/2
  AND/1 -> gate_enable_out/1

== system gm_interlock_deadtime/interlock_deadtime/EnableOutputModule_instance2 ==
  gate_delay_out : Inport  OutDataTypeStr=boolean  PortDimensions=1  SampleTime=1e-08
  enable : Inport  Port=2  OutDataTypeStr=boolean  PortDimensions=1  SampleTime=1e-08
  AND : Logic  AllPortsSameDT=off  OutDataTypeStr=boolean  SampleTime=1e-08
  gate_enable_out : Outport
  wires:
  AND/1 -> gate_enable_out/1
  enable/1 -> AND/2
  gate_delay_out/1 -> AND/1

== system gm_interlock_deadtime/interlock_deadtime/EnableOutputModule_instance3 ==
  gate_delay_out : Inport  OutDataTypeStr=boolean  PortDimensions=1  SampleTime=1e-08
  enable : Inport  Port=2  OutDataTypeStr=boolean  PortDimensions=1  SampleTime=1e-08
  AND : Logic  AllPortsSameDT=off  OutDataTypeStr=boolean  SampleTime=1e-08
  gate_enable_out : Outport
  wires:
  AND/1 -> gate_enable_out/1
  enable/1 -> AND/2
  gate_delay_out/1 -> AND/1

== system gm_interlock_deadtime/interlock_deadtime/EnableOutputModule_instance4 ==
  gate_delay_out : Inport  OutDataTypeStr=boolean  PortDimensions=1  SampleTime=1e-08
  enable : Inport  Port=2  OutDataTypeStr=boolean  PortDimensions=1  SampleTime=1e-08
  AND : Logic  AllPortsSameDT=off  OutDataTypeStr=boolean  SampleTime=1e-08
  gate_enable_out : Outport
  wires:
  AND/1 -> gate_enable_out/1
  enable/1 -> AND/2
  gate_delay_out/1 -> AND/1

== system gm_interlock_deadtime/interlock_deadtime/EnableOutputModule_instance5 ==
  gate_delay_out : Inport  OutDataTypeStr=boolean  PortDimensions=1  SampleTime=1e-08
  enable : Inport  Port=2  OutDataTypeStr=boolean  PortDimensions=1  SampleTime=1e-08
  AND : Logic  AllPortsSameDT=off  OutDataTypeStr=boolean  SampleTime=1e-08
  gate_enable_out : Outport
  wires:
  AND/1 -> gate_enable_out/1
  enable/1 -> AND/2
  gate_delay_out/1 -> AND/1

== system gm_interlock_deadtime/interlock_deadtime/EnableOutputModule_instance6 ==
  gate_delay_out : Inport  OutDataTypeStr=boolean  PortDimensions=1  SampleTime=1e-08
  enable : Inport  Port=2  OutDataTypeStr=boolean  PortDimensions=1  SampleTime=1e-08
  AND : Logic  AllPortsSameDT=off  OutDataTypeStr=boolean  SampleTime=1e-08
  gate_enable_out : Outport
  wires:
  AND/1 -> gate_enable_out/1
  enable/1 -> AND/2
  gate_delay_out/1 -> AND/1

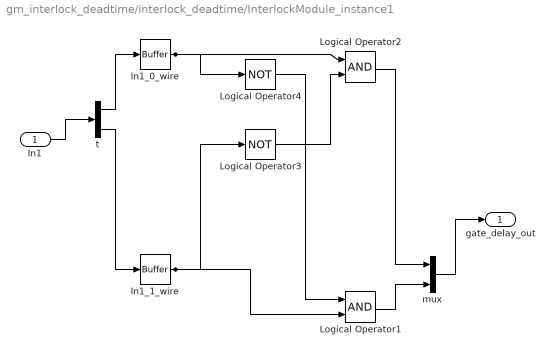
== system gm_interlock_deadtime/interlock_deadtime/InterlockModule_instance1 ==
  In1 : Inport  OutDataTypeStr=boolean  PortDimensions=[2]  SampleTime=1e-08
  In1_0_wire : hdlmdlgenlib/Buffer
      settings: SourceProductBaseCode=SL
  In1_1_wire : hdlmdlgenlib/Buffer
      settings: SourceProductBaseCode=SL
  Logical Operator1 : Logic  AllPortsSameDT=off  OutDataTypeStr=boolean  SampleTime=1e-08
  Logical Operator2 : Logic  AllPortsSameDT=off  OutDataTypeStr=boolean  SampleTime=1e-08
  Logical Operator3 : Logic  Operator=NOT  Inputs=1  AllPortsSameDT=off  OutDataTypeStr=boolean  SampleTime=1e-08
  Logical Operator4 : Logic  Operator=NOT  Inputs=1  AllPortsSameDT=off  OutDataTypeStr=boolean  SampleTime=1e-08
  mux : Mux  Inputs=2
  t : Demux  Outputs=2
  gate_delay_out : Outport
  wires:
  In1/1 -> t/1
  mux/1 -> gate_delay_out/1
  Logical Operator4/1 -> Logical Operator1/1
  Logical Operator3/1 -> Logical Operator2/2
  Logical Operator2/1 -> mux/1
  Logical Operator1/1 -> mux/2
  In1_0_wire/1 -> Logical Operator2/1, Logical Operator4/1
  In1_1_wire/1 -> Logical Operator1/2, Logical Operator3/1
  t/1 -> In1_0_wire/1
  t/2 -> In1_1_wire/1

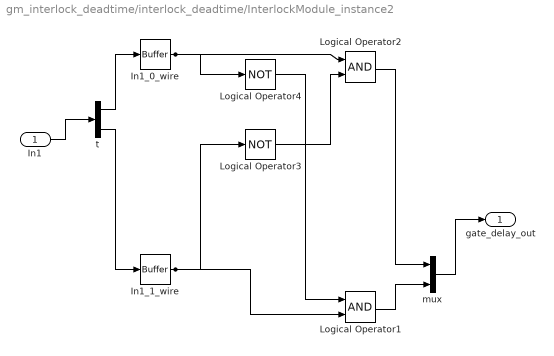
== system gm_interlock_deadtime/interlock_deadtime/InterlockModule_instance2 ==
  In1 : Inport  OutDataTypeStr=boolean  PortDimensions=[2]  SampleTime=1e-08
  In1_0_wire : hdlmdlgenlib/Buffer
      settings: SourceProductBaseCode=SL
  In1_1_wire : hdlmdlgenlib/Buffer
      settings: SourceProductBaseCode=SL
  Logical Operator1 : Logic  AllPortsSameDT=off  OutDataTypeStr=boolean  SampleTime=1e-08
  Logical Operator2 : Logic  AllPortsSameDT=off  OutDataTypeStr=boolean  SampleTime=1e-08
  Logical Operator3 : Logic  Operator=NOT  Inputs=1  AllPortsSameDT=off  OutDataTypeStr=boolean  SampleTime=1e-08
  Logical Operator4 : Logic  Operator=NOT  Inputs=1  AllPortsSameDT=off  OutDataTypeStr=boolean  SampleTime=1e-08
  mux : Mux  Inputs=2
  t : Demux  Outputs=2
  gate_delay_out : Outport
  wires:
  t/2 -> In1_1_wire/1
  t/1 -> In1_0_wire/1
  In1_1_wire/1 -> Logical Operator3/1, Logical Operator1/2
  In1_0_wire/1 -> Logical Operator4/1, Logical Operator2/1
  Logical Operator1/1 -> mux/2
  Logical Operator2/1 -> mux/1
  Logical Operator3/1 -> Logical Operator2/2
  Logical Operator4/1 -> Logical Operator1/1
  mux/1 -> gate_delay_out/1
  In1/1 -> t/1

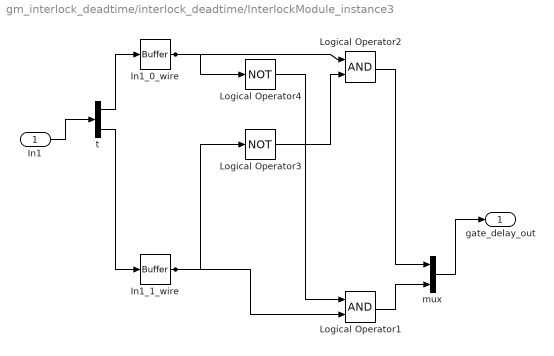
== system gm_interlock_deadtime/interlock_deadtime/InterlockModule_instance3 ==
  In1 : Inport  OutDataTypeStr=boolean  PortDimensions=[2]  SampleTime=1e-08
  In1_0_wire : hdlmdlgenlib/Buffer
      settings: SourceProductBaseCode=SL
  In1_1_wire : hdlmdlgenlib/Buffer
      settings: SourceProductBaseCode=SL
  Logical Operator1 : Logic  AllPortsSameDT=off  OutDataTypeStr=boolean  SampleTime=1e-08
  Logical Operator2 : Logic  AllPortsSameDT=off  OutDataTypeStr=boolean  SampleTime=1e-08
  Logical Operator3 : Logic  Operator=NOT  Inputs=1  AllPortsSameDT=off  OutDataTypeStr=boolean  SampleTime=1e-08
  Logical Operator4 : Logic  Operator=NOT  Inputs=1  AllPortsSameDT=off  OutDataTypeStr=boolean  SampleTime=1e-08
  mux : Mux  Inputs=2
  t : Demux  Outputs=2
  gate_delay_out : Outport
  wires:
  t/2 -> In1_1_wire/1
  t/1 -> In1_0_wire/1
  In1_1_wire/1 -> Logical Operator3/1, Logical Operator1/2
  In1_0_wire/1 -> Logical Operator4/1, Logical Operator2/1
  Logical Operator1/1 -> mux/2
  Logical Operator2/1 -> mux/1
  Logical Operator3/1 -> Logical Operator2/2
  Logical Operator4/1 -> Logical Operator1/1
  mux/1 -> gate_delay_out/1
  In1/1 -> t/1

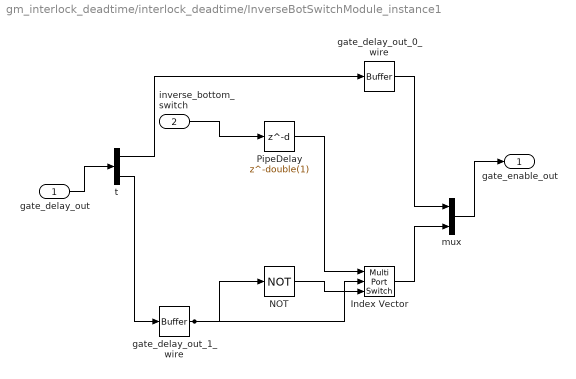
== system gm_interlock_deadtime/interlock_deadtime/InverseBotSwitchModule_instance1 ==
  gate_delay_out : Inport  OutDataTypeStr=boolean  PortDimensions=[2]  SampleTime=1e-08
  inverse_bottom_switch : Inport  Port=2  OutDataTypeStr=boolean  PortDimensions=1  SampleTime=1e-08
  Index Vector : MultiPortSwitch  DataPortOrder=Zero-based contiguous  Inputs=2  DiagnosticForDefault=None  zeroidx=on  SampleTime=1e-08
  NOT : Logic  Operator=NOT  Inputs=1  AllPortsSameDT=off  OutDataTypeStr=boolean  SampleTime=1e-08
  PipeDelay : Delay  DelayLength=double(1)  InitialCondition=0  SampleTime=1e-08
  gate_delay_out_0_wire : hdlmdlgenlib/Buffer
      settings: SourceProductBaseCode=SL
  gate_delay_out_1_wire : hdlmdlgenlib/Buffer
      settings: SourceProductBaseCode=SL
  mux : Mux  Inputs=2
  t : Demux  Outputs=2
  gate_enable_out : Outport
  wires:
  gate_delay_out/1 -> t/1
  inverse_bottom_switch/1 -> PipeDelay/1
  PipeDelay/1 -> Index Vector/1
  NOT/1 -> Index Vector/3
  mux/1 -> gate_enable_out/1
  Index Vector/1 -> mux/2
  gate_delay_out_0_wire/1 -> mux/1
  gate_delay_out_1_wire/1 -> Index Vector/2, NOT/1
  t/1 -> gate_delay_out_0_wire/1
  t/2 -> gate_delay_out_1_wire/1

== system gm_interlock_deadtime/interlock_deadtime/InverseBotSwitchModule_instance2 ==
  gate_delay_out : Inport  OutDataTypeStr=boolean  PortDimensions=[2]  SampleTime=1e-08
  inverse_bottom_switch : Inport  Port=2  OutDataTypeStr=boolean  PortDimensions=1  SampleTime=1e-08
  Index Vector : MultiPortSwitch  DataPortOrder=Zero-based contiguous  Inputs=2  DiagnosticForDefault=None  zeroidx=on  SampleTime=1e-08
  NOT : Logic  Operator=NOT  Inputs=1  AllPortsSameDT=off  OutDataTypeStr=boolean  SampleTime=1e-08
  PipeDelay : Delay  DelayLength=double(1)  InitialCondition=0  SampleTime=1e-08
  gate_delay_out_0_wire : hdlmdlgenlib/Buffer
      settings: SourceProductBaseCode=SL
  gate_delay_out_1_wire : hdlmdlgenlib/Buffer
      settings: SourceProductBaseCode=SL
  mux : Mux  Inputs=2
  t : Demux  Outputs=2
  gate_enable_out : Outport
  wires:
  t/2 -> gate_delay_out_1_wire/1
  t/1 -> gate_delay_out_0_wire/1
  gate_delay_out_1_wire/1 -> NOT/1, Index Vector/2
  gate_delay_out_0_wire/1 -> mux/1
  Index Vector/1 -> mux/2
  mux/1 -> gate_enable_out/1
  NOT/1 -> Index Vector/3
  PipeDelay/1 -> Index Vector/1
  inverse_bottom_switch/1 -> PipeDelay/1
  gate_delay_out/1 -> t/1

== system gm_interlock_deadtime/interlock_deadtime/InverseBotSwitchModule_instance3 ==
  gate_delay_out : Inport  OutDataTypeStr=boolean  PortDimensions=[2]  SampleTime=1e-08
  inverse_bottom_switch : Inport  Port=2  OutDataTypeStr=boolean  PortDimensions=1  SampleTime=1e-08
  Index Vector : MultiPortSwitch  DataPortOrder=Zero-based contiguous  Inputs=2  DiagnosticForDefault=None  zeroidx=on  SampleTime=1e-08
  NOT : Logic  Operator=NOT  Inputs=1  AllPortsSameDT=off  OutDataTypeStr=boolean  SampleTime=1e-08
  PipeDelay : Delay  DelayLength=double(1)  InitialCondition=0  SampleTime=1e-08
  gate_delay_out_0_wire : hdlmdlgenlib/Buffer
      settings: SourceProductBaseCode=SL
  gate_delay_out_1_wire : hdlmdlgenlib/Buffer
      settings: SourceProductBaseCode=SL
  mux : Mux  Inputs=2
  t : Demux  Outputs=2
  gate_enable_out : Outport
  wires:
  t/2 -> gate_delay_out_1_wire/1
  t/1 -> gate_delay_out_0_wire/1
  gate_delay_out_1_wire/1 -> NOT/1, Index Vector/2
  gate_delay_out_0_wire/1 -> mux/1
  Index Vector/1 -> mux/2
  mux/1 -> gate_enable_out/1
  NOT/1 -> Index Vector/3
  PipeDelay/1 -> Index Vector/1
  inverse_bottom_switch/1 -> PipeDelay/1
  gate_delay_out/1 -> t/1
